simulink model "PI_sim"  (R2018a)
settings: Solver=VariableStepAuto  StartTime=0.0  StopTime=100  RelTol=1e-3
values from neighbouring files (symbols this model uses):
  tmF = (1.2620*TTF(1))-(0.2620*TTF(3))    [Controlador_Flujo_PI - v1}.m]    (also in Controlador_Flujo_PI.m; Controlador_Flujo_PID.m; Controlador_Flujo_PID_tm.m; Controlador_Flujo_PI_VF.m)
undefined symbols (not defined in the file or in its folder): D1, den, N1, num
settings Model: Creator=Dell  LastModifiedBy=Dell

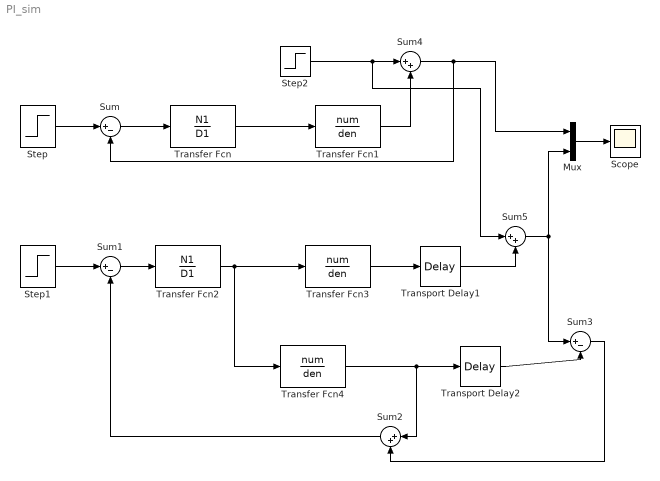
== system PI_sim ==
  Mux : Mux  Inputs=2
  Scope : Scope
  Step : Step  Time=0  SampleTime=0
  Step1 : Step  Time=0  SampleTime=0
  Step2 : Step  Time=30  After=0.4  SampleTime=0
  Sum : Sum  Inputs=|+-
  Sum1 : Sum  Inputs=|+-
  Sum2 : Sum  Inputs=|++
  Sum3 : Sum  Inputs=|+-
  Sum4 : Sum  Inputs=|++
  Sum5 : Sum  Inputs=|++
  Transfer Fcn : TransferFcn  Numerator=N1  Denominator=D1
  Transfer Fcn1 : TransferFcn  Numerator=num  Denominator=den
  Transfer Fcn2 : TransferFcn  Numerator=N1  Denominator=D1
  Transfer Fcn3 : TransferFcn  Numerator=num  Denominator=den
  Transfer Fcn4 : TransferFcn  Numerator=num  Denominator=den
  Transport Delay1 : TransportDelay  DelayTime=tmF
  Transport Delay2 : TransportDelay  DelayTime=tmF
  wires:
  Transfer Fcn/1 -> Transfer Fcn1/1
  Step/1 -> Sum/1
  Sum/1 -> Transfer Fcn/1
  Mux/1 -> Scope/1
  Transfer Fcn3/1 -> Transport Delay1/1
  Transfer Fcn2/1 -> Transfer Fcn3/1, Transfer Fcn4/1
  Sum1/1 -> Transfer Fcn2/1
  Step1/1 -> Sum1/1
  Transfer Fcn4/1 -> Transport Delay2/1, Sum2/1
  Sum2/1 -> Sum1/2
  Transport Delay2/1 -> Sum3/2
  Sum3/1 -> Sum2/2
  Step2/1 -> Sum5/1, Sum4/1
  Transfer Fcn1/1 -> Sum4/2
  Sum4/1 -> Sum/2, Mux/1
  Transport Delay1/1 -> Sum5/2
  Sum5/1 -> Sum3/1, Mux/2
